simulink model "ArduinoModel"  (R2014a)
settings: Solver=ode3  SolverMode=SingleTasking  StartTime=0.0  StopTime=Inf  FixedStep=0.1  RelTol=1e-3
PostLoadFcn:
  | loadRobotParameters
  | 
  | allotedRunTime = 3*60; % [sec] Time allowed for run
  | 
  | % starting parameters
  | % The timer starts once the robot has moved a certain distance from the
  | % starting point
  | startPos = [50 50]; % [cm]
  | startingRadius = 10; % [cm]
  | 
  | % Target parameters
  | targetBoundaryRadius = 7; % [cm] radius considered at location
  | statTimeReq = 2.5; % [sec] minimum time robot must be at location
InitFcn:
  | close('all','force');
StartFcn:
  | %reset(SimDisplay.getInstance());
undefined symbols (not defined in the file): AxleLength, EncRes, lcam, pcam, SitesPositions, Ts, WheelRadius
libraries: arduinodue_drivers x6, arduinolib x5, simulink x1
CloseFcn:
  | close('all','force');
settings Model: SimulationMode=external  PauseTimes=14  ExtModeTrigDuration=2  Creator=gpacitti  LastModifiedBy=odufour
settings DataIOCC: SignalLoggingSaveFormat=ModelDataLogs  SaveOutput=off  SignalLogging=off  DSMLogging=off  SaveTime=off
settings OptimizationCC: ExpressionDepthLimit=2147483647  OptimizeModelRefInitCode=on  LifeSpan=Inf
settings DebuggingCC: UnderspecifiedInitializationDetection=Classic  SolverPrmCheckMsg=none  InheritedTsInSrcMsg=none  MultiTaskDSMMsg=warning  MultiTaskCondExecSysMsg=none  ParameterPrecisionLossMsg=none  StateNameClashWarn=warning
settings HardwareCC: ProdLargestAtomicInteger=Long  ProdLargestAtomicFloat=Double  ProdEndianess=LittleEndian  ProdHWDeviceType=ARM Compatible->ARM Cortex
settings RTWCC: SystemTargetFile=realtime.tlc  GenerateMakefile=off  TemplateMakefile=realtime.tmf  Description=Run on Target Hardware  RTWVerbose=off  ProcessScript=realtime_make_rtw_hook  IncludeERTFirstTime=on
settings CodeAppCC: CustomSymbolStrType=$N$R$M  InternalIdentifier=Classic
settings STFCustomTargetCC: TargetLibSuffix=.a  GenerateSampleERTMain=on  ConcurrentExecutionCompliant=off  GeneratePreprocessorConditionals=Use local settings  ERTCustomFileBanners=on  SupportNonInlinedSFcns=off  SupportVariableSizeSignals=on  MATLABClassNameForMDSCustomization=Simulink.SoftwareTarget.ERTCustomization  GRTInterface=off  SystemTargetFile=realtime.tlc
settings ERTTargetCC: CombineOutputUpdateFcns=off  SupportContinuousTime=on  SupportVariableSizeSignals=on  ExtMode=on  ExtModeTransport=3  ExtModeMexFile=ext_serial_win32_comm  ExtModeMexArgs=0 17 115200 30  ERTSrcFileBannerTemplate=realtime_code_template.cgt  ERTHdrFileBannerTemplate=realtime_code_template.cgt  ERTDataSrcFileTemplate=realtime_code_template.cgt  ERTDataHdrFileTemplate=realtime_code_template.cgt  ERTCustomFileTemplate=realtime_file_process.tlc
settings ConfigComp: Description=Design Verifier Custom Configuration Component  DVMaxTestCaseSteps=500  DVTestSuiteOptimization=CombinedObjectives (Nonlinear Extended)

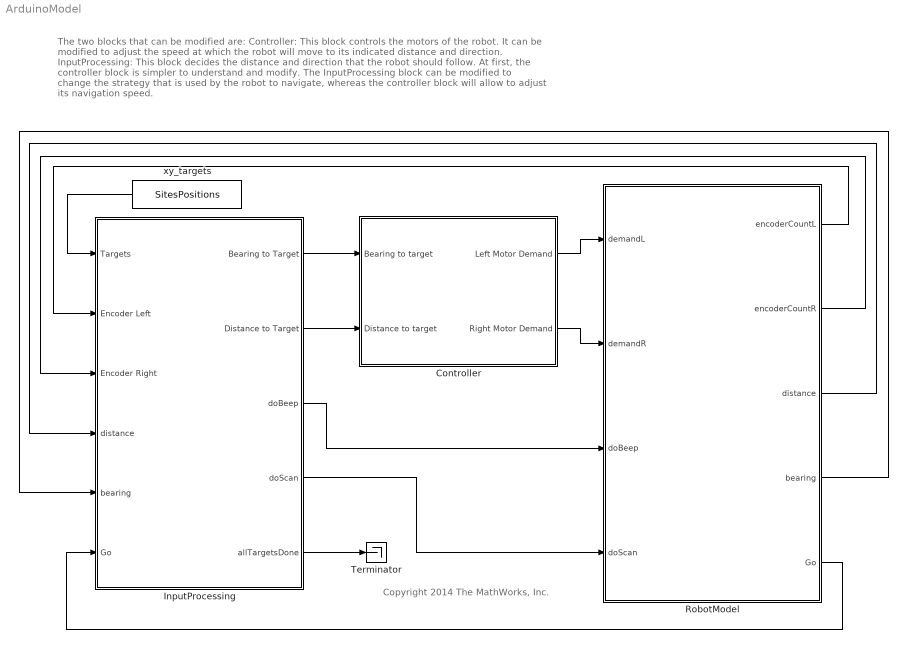
== system ArduinoModel ==
  note: Copyright 2014 The MathWorks, Inc.
  note: The two blocks that can be modified are:
      | Controller: This block controls the motors of the robot. It can be modified to adjust the speed at which the robot will move to its indicated distance and direction.
      | InputProcessing: This block decides the distance and direction that the robot should follow.
      |
      | At first, the controller block is simpler to understand and modify.
      | The InputProcessing block can be modified to change the strategy that is used by the robot to navigate, whereas the controller block will allow to adjust its navigation speed.
  Controller : Subsystem  TreatAsAtomicUnit=on
      mask Display: image('Arduino_Mega_2560.jpg',[0.75/2,0.3,0.25,0.4]);
  InputProcessing : Subsystem
      mask Display: image('Arduino_Mega_2560.jpg',[0.75/2,0.3,0.25,0.3]);
  RobotModel : Subsystem
      mask Display: image('robot_3d.jpg',[0.25,0.35,0.45,0.25]);
  Terminator : Terminator
  xy_targets : Constant  Value=SitesPositions  OutDataTypeStr=single
  wires:
  RobotModel/2(encoderCountR) -> InputProcessing/3(Encoder Right)
  RobotModel/1(encoderCountL) -> InputProcessing/2(Encoder Left)
  xy_targets/1 -> InputProcessing/1(Targets)
  InputProcessing/2(Distance to Target) -> Controller/2(Distance to target)
  InputProcessing/1(Bearing to Target) -> Controller/1(Bearing to target)
  Controller/1(Left Motor Demand) -> RobotModel/1(demandL)
  Controller/2(Right Motor Demand) -> RobotModel/2(demandR)
  RobotModel/3(distance) -> InputProcessing/4(distance)
  RobotModel/4(bearing) -> InputProcessing/5(bearing)
  RobotModel/5(Go) -> InputProcessing/6(Go)
  InputProcessing/5(allTargetsDone) -> Terminator/1
  InputProcessing/4(doScan) -> RobotModel/4(doScan)
  InputProcessing/3(doBeep) -> RobotModel/3(doBeep)

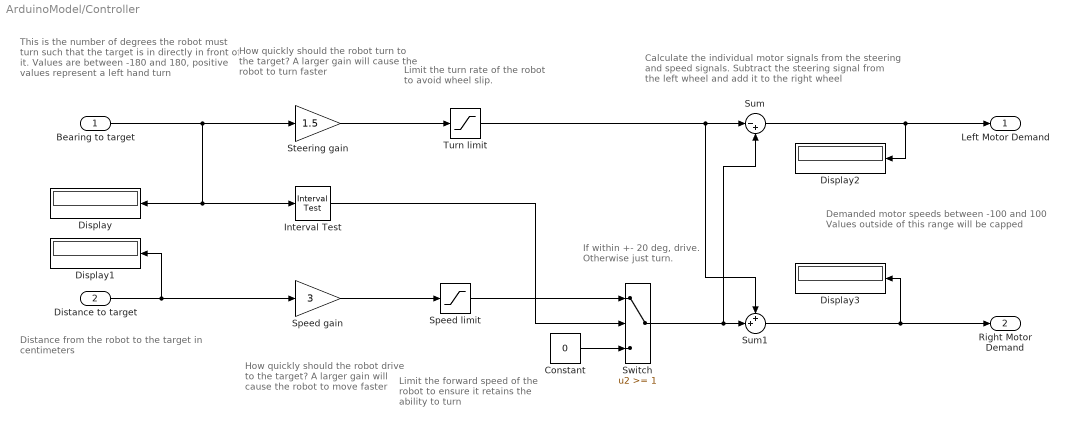
== system ArduinoModel/Controller ==
  note: This is the number of degrees the robot
      | must turn such that the target is in directly
      | in front of it.
      | Values are between -180 and 180,
      | positive values represent a left hand turn
  note: Distance from the robot to the target
      | in centimeters
  note: Demanded motor speeds between -100 and 100
      | Values outside of this range will be capped
  note: How quickly should the robot turn
      | to the target? A larger gain will
      |  cause the robot to turn faster
  note: How quickly should the robot
      | drive to the target? A larger gain
      | will cause the robot to move
      | faster
  note: Limit the forward speed of the
      | robot to ensure it retains the
      | ability to turn
  note: Calculate the individual motor signals from the
      | steering and speed signals. Subtract the steering
      | signal from the left wheel and add it to the right
      | wheel
  note: If within +- 20 deg, drive.
      | Otherwise just turn.
  note: Limit the turn rate of the
      | robot to avoid wheel slip.
  Bearing to target : Inport  OutDataTypeStr=single
  Distance to target : Inport  Port=2  PortDimensions=1  SampleTime=Ts
  Constant : Constant  Value=0  OutDataTypeStr=single
  Display{,1..3} (4 alike) : Display
  Interval Test : simulink/Logic and Bit Operations/Interval Test  IntervalClosedRight=on  uplimit=25  IntervalClosedLeft=on  lowlimit=-25  OutDataTypeStr=boolean
      settings: AttributesFormatString=|
      | Upper = %<uplimit>
      | Lower = %<lowlimit>
  Speed gain : Gain  Gain=3
  Speed limit : Saturate  UpperLimit=50  LowerLimit=0
      settings: AttributesFormatString=|
      | Upper = %<UpperLimit>
      | Lower = %<LowerLimit>
  Steering gain : Gain  Gain=1.5
  Sum : Sum  Inputs=|-+
  Sum1 : Sum  Inputs=++|
  Switch : Switch  Threshold=1
  Turn limit : Saturate  UpperLimit=50  LowerLimit=-50
      settings: AttributesFormatString=|
      | Upper = %<UpperLimit>
      | Lower = %<LowerLimit>
  Left Motor Demand : Outport  OutDataTypeStr=single
  Right Motor Demand : Outport  Port=2  OutDataTypeStr=single
  wires:
  Speed limit/1 -> Switch/1
  Turn limit/1 -> Sum1/1, Sum/1
  Constant/1 -> Switch/3
  Interval Test/1 -> Switch/2
  Switch/1 -> Sum1/2, Sum/2
  Sum/1 -> Display2/1, Left Motor Demand/1
  Sum1/1 -> Display3/1, Right Motor Demand/1
  Steering gain/1 -> Turn limit/1
  Distance to target/1 -> Speed gain/1, Display1/1
  Speed gain/1 -> Speed limit/1
  Bearing to target/1 -> Interval Test/1, Display/1, Steering gain/1

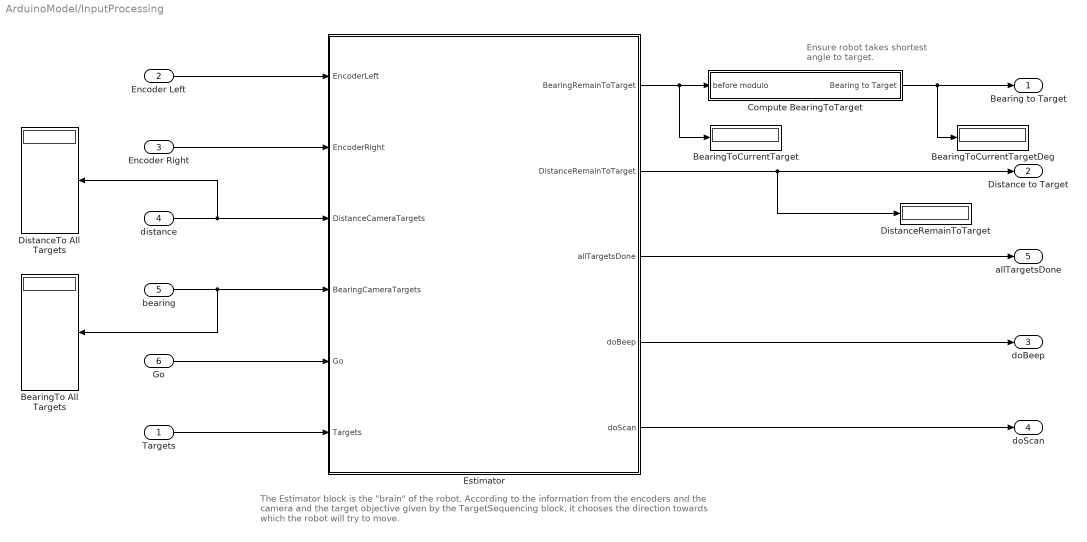
== system ArduinoModel/InputProcessing ==
  note: The Estimator block is the "brain" of the robot. According to the information from the encoders and the camera and the
      | target objective given by the TargetSequencing block, it chooses the direction towards which the robot will try to move.
  note: Ensure robot takes shortest
      | angle to target.
  Targets : Inport
  Encoder Left : Inport  Port=2
  Encoder Right : Inport  Port=3
  distance : Inport  Port=4
  bearing : Inport  Port=5
  Go : Inport  Port=6
  BearingTo All Targets : Display
  BearingToCurrentTarget : Display
  BearingToCurrentTargetDeg : Display
  Compute BearingToTarget : Subsystem
  DistanceRemainToTarget : Display
  DistanceTo All Targets : Display
  Estimator : Stateflow chart  TreatAsAtomicUnit=on
  Bearing to Target : Outport  SampleTime=Ts
  Distance to Target : Outport  Port=2
  doBeep : Outport  Port=3
  doScan : Outport  Port=4
  allTargetsDone : Outport  Port=5
  wires:
  distance/1 -> DistanceTo All Targets/1, Estimator/3(DistanceCameraTargets)
  bearing/1 -> BearingTo All Targets/1, Estimator/4(BearingCameraTargets)
  Compute BearingToTarget/1(Bearing to Target) -> BearingToCurrentTargetDeg/1, Bearing to Target/1
  Estimator/2(DistanceRemainToTarget) -> DistanceRemainToTarget/1, Distance to Target/1
  Estimator/1(BearingRemainToTarget) -> Compute BearingToTarget/1(before modulo), BearingToCurrentTarget/1
  Encoder Right/1 -> Estimator/2(EncoderRight)
  Encoder Left/1 -> Estimator/1(EncoderLeft)
  Targets/1 -> Estimator/6(Targets)
  Go/1 -> Estimator/5(Go)
  Estimator/3(allTargetsDone) -> allTargetsDone/1
  Estimator/4(doBeep) -> doBeep/1
  Estimator/5(doScan) -> doScan/1

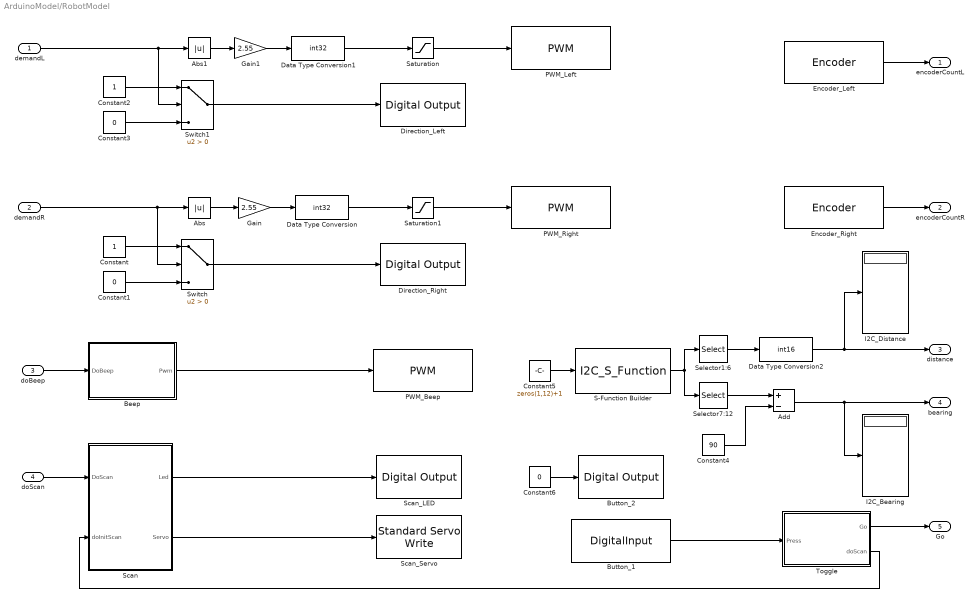
== system ArduinoModel/RobotModel ==
  demandL : Inport  SampleTime=0
  demandR : Inport  Port=2  SampleTime=0
  doBeep : Inport  Port=3  SampleTime=0
  doScan : Inport  Port=4  SampleTime=0
  Abs : Abs
  Abs1 : Abs
  Add : Sum  Inputs=+-  OutDataTypeStr=int8
  Beep : Stateflow chart  TreatAsAtomicUnit=on
  Button_1 : arduinodue_drivers/DigitalInput  pinNumber=14  isPullUp=on
  Button_2 : arduinolib/Digital Output  pinNumber=15
  Constant : Constant  OutDataTypeStr=uint8
  Constant1 : Constant  Value=0  OutDataTypeStr=uint8
  Constant2 : Constant  OutDataTypeStr=uint8
  Constant3 : Constant  Value=0  OutDataTypeStr=uint8
  Constant4 : Constant  Value=90  OutDataTypeStr=uint8
  Constant5 : Constant  Value=zeros(1,12)+1  OutDataTypeStr=uint8
  Constant6 : Constant  Value=0  OutDataTypeStr=uint8
  Data Type Conversion : DataTypeConversion  OutDataTypeStr=int32  SaturateOnIntegerOverflow=on
  Data Type Conversion1 : DataTypeConversion  OutDataTypeStr=int32  SaturateOnIntegerOverflow=on
  Data Type Conversion2 : DataTypeConversion  OutDataTypeStr=int16  SaturateOnIntegerOverflow=on
  Direction_Left : arduinolib/Digital Output  pinNumber=7
  Direction_Right : arduinolib/Digital Output  pinNumber=4
  Encoder_Left : arduinodue_drivers/Encoder  pinA=19  pinB=18
  Encoder_Right : arduinodue_drivers/Encoder  pinA=16  pinB=17
  Gain : Gain  Gain=2.55
  Gain1 : Gain  Gain=2.55
  I2C_Bearing : Display
  I2C_Distance : Display
  PWM_Beep : arduinodue_drivers/PWM  pinNumber=10
  PWM_Left : arduinodue_drivers/PWM  pinNumber=6
  PWM_Right : arduinodue_drivers/PWM  pinNumber=5
  S-Function Builder : S-Function  InitFcn=try, set_param(gcb,'FunctionName','I2C_S_Function'), end  FunctionName=I2C_S_Function  Parameters=uint8(1)  SFunctionModules=I2C_S_Function_wrapper  EnableBusSupport=off  mask(S-Function Builder){}
      mask help: Simulink:masks:SFunctionBuilder_MD
      mask init:
      | val = [[.9  0.75 0.75 1 1 .9 .9 1]',[1 1 0.75 0.75 .9 .9 1 .9]'];try , sys = get_param(gcb,'SfunBuilderFcnName');if isempty(sys), sys = get_param(gcb,'FunctionName'); end,catch, sys = get_param(gcb,'FunctionName'); end
      settings: CopyFcn=set_param(gcbh,'LinkStatus','none')  PreSaveFcn=try, set_param(gcb,'FunctionName','I2C_S_Function'), end  OpenFcn=sfunctionwizard(gcbh)
      mask Display: plot(val(:,1),val(:,2)),disp(sys), port_label('input',1,'u0'), port_label('output',1,'y0')
  Saturation : Saturate  UpperLimit=255  LowerLimit=0
  Saturation1 : Saturate  UpperLimit=255  LowerLimit=0
  Scan : Stateflow chart  TreatAsAtomicUnit=on
  Scan_LED : arduinolib/Digital Output  pinNumber=23
  Scan_Servo : arduinolib/Standard Servo Write  pinNumber=22
  Selector1:6 : Selector  InputPortWidth=12  Indices=[1:6]
  Selector7:12 : Selector  InputPortWidth=12  Indices=[7:12]
  Switch : Switch  Criteria=u2 > Threshold
  Switch1 : Switch  Criteria=u2 > Threshold
  Toggle : Stateflow chart  TreatAsAtomicUnit=on
  encoderCountL : Outport  OutDataTypeStr=int32
  encoderCountR : Outport  Port=2  OutDataTypeStr=int32
  distance : Outport  Port=3
  bearing : Outport  Port=4
  Go : Outport  Port=5
  wires:
  Encoder_Right/1 -> encoderCountR/1
  Encoder_Left/1 -> encoderCountL/1
  Abs/1 -> Gain/1
  Gain/1 -> Data Type Conversion/1
  Data Type Conversion/1 -> Saturation1/1
  Constant/1 -> Switch/1
  Constant1/1 -> Switch/3
  Switch/1 -> Direction_Right/1
  Abs1/1 -> Gain1/1
  Gain1/1 -> Data Type Conversion1/1
  Data Type Conversion1/1 -> Saturation/1
  Constant2/1 -> Switch1/1
  Constant3/1 -> Switch1/3
  Switch1/1 -> Direction_Left/1
  Data Type Conversion2/1 -> distance/1, I2C_Distance/1
  Add/1 -> I2C_Bearing/1, bearing/1
  demandR/1 -> Switch/2, Abs/1
  demandL/1 -> Switch1/2, Abs1/1
  Toggle/1(Go) -> Go/1
  S-Function Builder/1 -> Selector7:12/1, Selector1:6/1
  Selector7:12/1 -> Add/1
  Constant4/1 -> Add/2
  Selector1:6/1 -> Data Type Conversion2/1
  doScan/1 -> Scan/1(DoScan)
  doBeep/1 -> Beep/1(DoBeep)
  Beep/1(Pwm) -> PWM_Beep/1
  Scan/2(Servo) -> Scan_Servo/1
  Saturation/1 -> PWM_Left/1
  Saturation1/1 -> PWM_Right/1
  Constant5/1 -> S-Function Builder/1
  Constant6/1 -> Button_2/1
  Scan/1(Led) -> Scan_LED/1
  Button_1/1 -> Toggle/1(Press)
  Toggle/2(doScan) -> Scan/2(doInitScan)

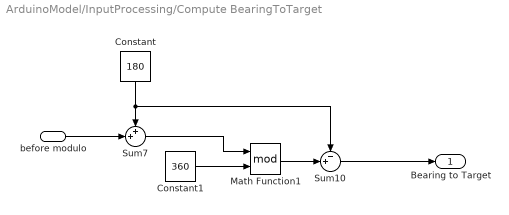
== system ArduinoModel/InputProcessing/Compute BearingToTarget ==
  before modulo : Inport
  Constant : Constant  Value=180  OutDataTypeStr=Inherit: Inherit via back propagation
  Constant1 : Constant  Value=360  OutDataTypeStr=Inherit: Inherit via back propagation
  Math Function1 : Math  Operator=mod  SaturateOnIntegerOverflow=on
  Sum10 : Sum  Inputs=-+|
  Sum7 : Sum  Inputs=++|
  Bearing to Target : Outport  SampleTime=Ts
  wires:
  before modulo/1 -> Sum7/2
  Sum10/1 -> Bearing to Target/1
  Math Function1/1 -> Sum10/2
  Constant1/1 -> Math Function1/2
  Sum7/1 -> Math Function1/1
  Constant/1 -> Sum10/1, Sum7/1

== stateflow chart ArduinoModel/RobotModel/Scan ==
  state Init
    entry: Servo = uint8(5);
  state Move_servo
    entry:
    Servo = uint8(60);
    during:
    if (mod(Servo,5) == 0)
    Led = uint8(1);
    else
    Led= uint8(0);
    end
    Servo = Servo + 2;
  (default) -> Init
  Init -> Move_servo [order 2] : [doInitScan]
  Init -> Move_servo [order 1] : [DoScan == true]
  Move_servo -> Init : [Servo == 120]
  data: DoScan input boolean; Led output uint8; Servo output uint8; doInitScan input

== stateflow chart ArduinoModel/InputProcessing/Estimator ==
  state Standby
    entry:
    %Init
    doBeep = false;doScan = false;
    encoder_left_prev_target = int32(0);
    encoder_right_prev_target = int32(0);
    ind = uint8(0);
    CurrentDistance = single(0);
    prev_target = single(startPos);
    prev_bearing = single(0);
    TargetIndex = uint8(0);
    allTargetsDone = false;
  state Running
    state Next_Target
      entry:
      doScan = false;
      TargetIndex = TargetIndex + 1;
      %Calc relative distance to next target
      DistanceToTarget = norm(Targets(TargetIndex,1:2)-prev_target);
      %Calc relative bearing to next target
      BearingToTarget = atan2d(Targets(TargetIndex,2)-prev_target(2),...
      Targets(TargetIndex,1)-prev_target(1)) - prev_bearing;
      %Save values for relative moves
      prev_target = Targets(TargetIndex,1:2);
      prev_bearing = prev_bearing + BearingToTarget;
      encoder_left_prev_target = EncoderLeft;
      encoder_right_prev_target = EncoderRight;
      DistanceRemainToTarget = DistanceToTarget;
      BearingRemainToTarget = BearingToTarget;
    state Apply_camera_correction
      entry:
      %Find the closest match between seen targets and current destination
      TargetFound = uint8(0);
      dist_remaining = int16(DistanceRemainToTarget);
      for ind=1:uint8(length(DistanceCameraTargets))
      if(DistanceCameraTargets(ind) ~= 0 )
      if(abs(DistanceCameraTargets(ind) - dist_remaining) < 15)
      if (TargetFound == 0 || abs(DistanceCameraTargets(TargetFound) -  ...
      dist_remaining) > abs(DistanceCameraTargets(ind) - dist_remaining))
      TargetFound = uint8(ind);
      end
      end
      end
      end
      %If a target is found update the distance and bearing from the camera
      if ( TargetFound ~= 0 )
      doBeep = true;
      DistanceToTarget = single(DistanceCameraTargets(TargetFound));
      BearingToTarget = single(BearingCameraTargets(TargetFound))/2;
      encoder_left_prev_target = EncoderLeft;
      encoder_right_prev_target = EncoderRight;
      end
    state Wait_for_scoring
      entry:
      DistanceRemainToTarget = single(0);
      doScan = true;
    state Calc_next_robot_move
      entry,during:
      doBeep = false;
      %Calc the new trajectory based on what has already been done
      dL = single(EncoderLeft - encoder_left_prev_target) * 2 * WheelRadius * pi / EncRes;
      dR = single(EncoderRight - encoder_right_prev_target) * 2 * WheelRadius * pi / EncRes;
      CurrentDistance = ((dL + dR)/2);
      CurrentBearing = single(((dR - dL)*180) / (AxleLength*1.01*pi));
      DistanceRemainToTarget = DistanceToTarget - CurrentDistance;
      BearingRemainToTarget = BearingToTarget - CurrentBearing;
    (default) -> Next_Target
    Next_Target -> Calc_next_robot_move
    Wait_for_scoring -> Next_Target : after(3,sec)
    Calc_next_robot_move -> Wait_for_scoring [order 1] : [DistanceRemainToTarget < 7]
    Apply_camera_correction -> Calc_next_robot_move
    Calc_next_robot_move -> Apply_camera_correction [order 2] : [CurrentDistance > 5 && DistanceRemainToTarget > pcam(1)-5]
  state All_targets_done
    entry:
    DistanceRemainToTarget = single(0);
    doScan = true;
  state Finished
    entry:
    allTargetsDone = true;
    doScan = false;
  (default) -> Standby
  Standby -> Running : [Go == true]
  Running -> All_targets_done : [DistanceRemainToTarget < 7 && TargetIndex >= length(Targets) ]
  All_targets_done -> Finished : after(3,sec)
  data: BearingRemainToTarget output single size=1; TargetIndex local uint8 size=1 =0; EncoderLeft input int32 size=1; EncoderRight input int32 size=1; DistanceRemainToTarget output single size=1; DistanceCameraTargets input int16; TargetFound local uint8 size=1; BearingCameraTargets input int8; AxleLength parameter single size=1; WheelRadius parameter single size=1; EncRes parameter single size=1; encoder_right_prev_target local int32; ind local uint8; dR local single; dL local single; CurrentDistance local single; CurrentBearing local single; dist_remaining local int16; encoder_left_prev_target local int32; Go input boolean; startPos parameter; Targets input single; prev_target local single; prev_bearing local single; BearingToTarget local single; DistanceToTarget local single; allTargetsDone output boolean; doBeep output boolean; doScan output boolean; pcam parameter; lcam parameter

== stateflow chart ArduinoModel/RobotModel/Toggle ==
  state OFF
    entry:
    Go = false;
    doScan = false;
  state ON
    entry:
    Go = true;
    doScan = false;
  state Wait
    entry: doScan = true;
  (default) -> OFF
  OFF -> Wait : [Press == 0]
  Wait -> ON : after(3,sec)
  data: Press input; Go output; doScan output

== stateflow chart ArduinoModel/RobotModel/Beep ==
  state Init
    entry:
    Pwm = int32(0);
  state Beep_on
    entry:
    Pwm = int32(50);
  state Beep_off
    entry:
    Pwm = int32(0);
  (default) -> Init
  Beep_on -> Beep_off : after(0.1,sec)
  Init -> Beep_on : [DoBeep == true]
  Beep_off -> Init : after(0.1,sec)
  data: DoBeep input boolean; Pwm output int32
